simulink model "coherentDemodulator"  (R2024a)
settings: Solver=VariableStepAuto  StartTime=0.0  StopTime=10.0  RelTol=1e-3
settings Model: Creator=prath  LastModifiedBy=prath

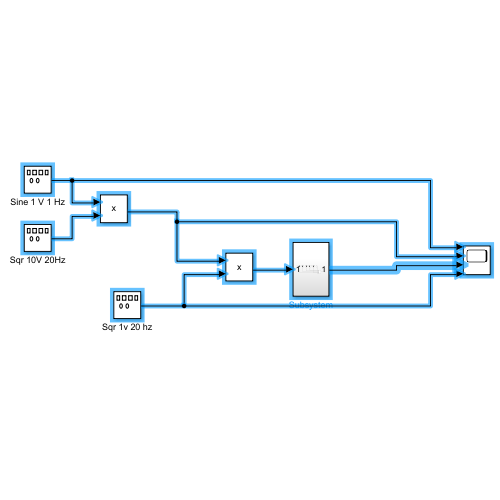
[thumbnail: Simulink's stored preview of the top-level diagram]
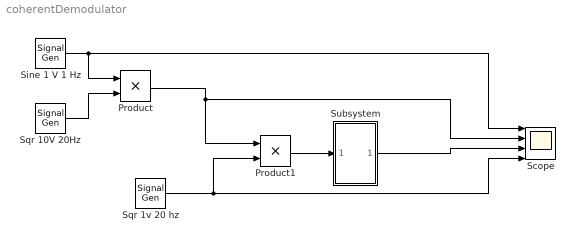
== system coherentDemodulator ==
  Product : Product
  Product1 : Product
  Scope : Scope  NumInputPorts=4
  Sine 1 V 1 Hz : SignalGenerator  Units=rad/sec  VectorParams1D=off
  Sqr 10V 20Hz : SignalGenerator  WaveForm=square  Amplitude=10  Frequency=20  Units=rad/sec  VectorParams1D=off
  Sqr 1v 20 hz : SignalGenerator  WaveForm=square  Frequency=20  Units=rad/sec
  Subsystem : Subsystem
  wires:
  Product1/1 -> Subsystem/1(In1)
  Product/1 -> Product1/1, Scope/2
  Sqr 10V 20Hz/1 -> Product/2
  Sqr 1v 20 hz/1 -> Scope/4, Product1/2
  Sine 1 V 1 Hz/1 -> Scope/1, Product/1
  Subsystem/1(Out1) -> Scope/3

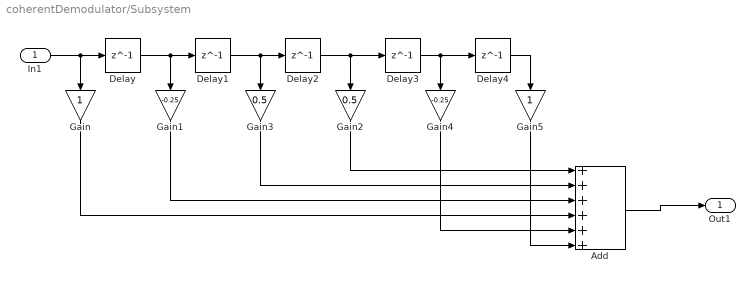
== system coherentDemodulator/Subsystem ==
  In1 : Inport
  Add : Sum  Inputs=++++++
  Delay{,1..4} (5 alike) : Delay  DelayLength=1
  Gain : Gain
  Gain1 : Gain  Gain=-0.25
  Gain2 : Gain  Gain=0.5
  Gain3 : Gain  Gain=0.5
  Gain4 : Gain  Gain=-0.25
  Gain5 : Gain
  Out1 : Outport
  wires:
  Delay3/1 -> Delay4/1, Gain4/1
  Delay1/1 -> Delay2/1, Gain3/1
  Gain2/1 -> Add/1
  Gain3/1 -> Add/2
  Delay2/1 -> Delay3/1, Gain2/1
  Delay/1 -> Delay1/1, Gain1/1
  In1/1 -> Gain/1, Delay/1
  Gain4/1 -> Add/5
  Delay4/1 -> Gain5/1
  Gain5/1 -> Add/6
  Gain1/1 -> Add/3
  Gain/1 -> Add/4
  Add/1 -> Out1/1
